simulink model "Lab1_DynamicDecoupledControllers"  (R2019a)
settings: Solver=VariableStepAuto  StartTime=0.0  StopTime=10.0  RelTol=1e-3
libraries: cstblocks x2
settings Model: Creator=emma  LastModifiedBy=emma

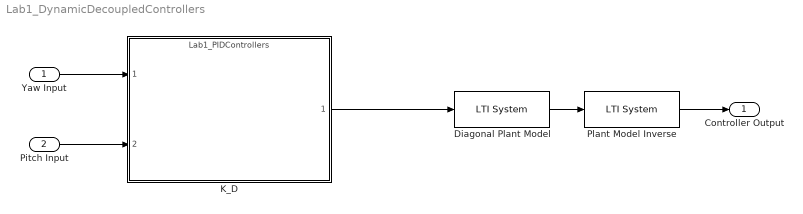
== system Lab1_DynamicDecoupledControllers ==
  Yaw Input : Inport
  Pitch Input : Inport  Port=2
  Diagonal Plant Model : cstblocks/LTI System  sys=Gd  IC=[]
  K_D : ModelReference  ModelNameDialog=Lab1_PIDControllers.slx  SimulationMode=Normal  ModelReferenceVersion=1.2
  Plant Model Inverse : cstblocks/LTI System  sys=Gm_inv  IC=[]
  Controller Output : Outport
  wires:
  K_D/1 -> Diagonal Plant Model/1
  Diagonal Plant Model/1 -> Plant Model Inverse/1
  Pitch Input/1 -> K_D/2
  Yaw Input/1 -> K_D/1
  Plant Model Inverse/1 -> Controller Output/1
